simulink model "mainV03_52"  (R2016b)
settings: Solver=FixedStepAuto  StartTime=0.0  StopTime=inf  FixedStep=Ts  MaxStep=0.2  RelTol=1e-2
undefined symbols (not defined in the file): checks, datetime, decyear, delta_e, deltae_degrees, deltafl_degrees, deltafr_degrees, deltar_degrees, deltat_1, deltat_2, deltat_3, deltat_4, deltat_5, Earth, F, ft, groundReaction, initialValues, juliandate, LD, leapyear, Light, m, MIL, Newton, Raphson, s, sigbuilder_block, Ts, WGS84
libraries: simulink x27, aerolibutil x17, aerolibtransform2 x12, aerolibasang x5, aerolib6dofsys x5, aerolib6dof2 x4, aerolibwind2 x3, aerolibbdyn x3, aerolibconvert2 x3, aerolibactuator x2, aerolibgravity2 x2, aerolibnav x2
(part 3 of 6)

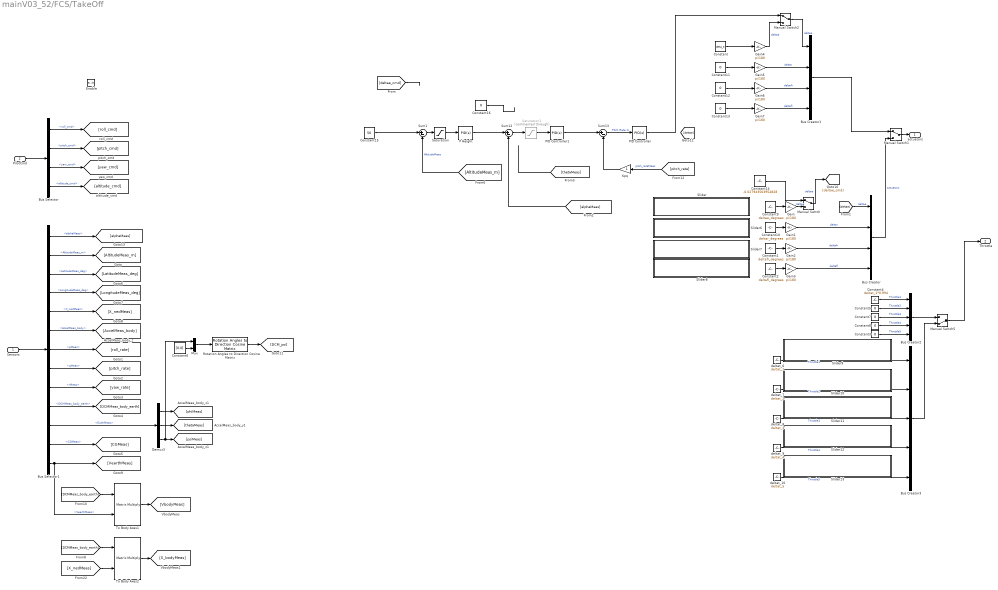
== system mainV03_52/FCS/TakeOff ==
  Sensors : Inport  OutDataTypeStr=Bus: SensorsBus
  PilotCmd : Inport  Port=2  OutDataTypeStr=Bus: CommandBus
  Enable : EnablePort
  Bus Creator : BusCreator  Inputs='deltae','deltar','deltafr','deltafl'  OutDataTypeStr=Bus: ActuatorsBus  NonVirtualBus=on
  Bus Creator1 : BusCreator  Inputs='deltae','deltar','deltafr','deltafl'  OutDataTypeStr=Bus: ActuatorsBus  NonVirtualBus=on
  Bus Creator2 : BusCreator  Inputs='Throttle1','Throttle2','Throttle3','Throttle4','Throttle5'  OutDataTypeStr=Bus: ThrottleBus  NonVirtualBus=on
  Bus Creator3 : BusCreator  Inputs='Throttle1','Throttle2','Throttle3','Throttle4','Throttle5'  OutDataTypeStr=Bus: ThrottleBus  NonVirtualBus=on
  Bus Selector : BusSelector  OutputSignals=roll_cmd,pitch_cmd,yaw_cmd,altitude_cmd
  Bus Selector1 : BusSelector  OutputSignals=alphaMeas,LLAMeas.AltitudeMeas_m,LLAMeas.LatitudeMeas_deg,LLAMeas.LongitudeMeas_deg,X_nedMeas,AccelMeas_body,OmegaMeas_body.pMeas,OmegaMeas_body.qMeas,OmegaMeas_body.rMeas,DCMMeas_body_earth,EulerMeas,CGMeas,VearthMeas
  Constant : Constant  Value=delta_e
  Constant1 : Constant  Value=deltafr_degrees
  Constant10 : Constant  Value=deltar_degrees
  Constant{3,5,7..8,11..13,16} (8 alike) : Constant  Value=0
  Constant14 : Constant  Value=-0.027943563954828
  Constant15 : Constant  Value=50
  Constant2 : Constant  Value=deltafl_degrees
  Constant4 : Constant  Value=deltat_1*0.994
  Constant6 : Constant  Value=[0,0]
  Constant9 : Constant  Value=deltae_degrees
  Demux3 : Demux  Outputs=3
  Gain{,1..7} (8 alike) : Gain  Gain=pi/180
  Kpq : Gain
  Manual Switch : ManualSwitch
  Manual Switch1 : ManualSwitch
  Manual Switch2 : ManualSwitch
  Manual Switch5 : ManualSwitch  CurrentSetting=0
  Mux : Mux  Inputs=2
  P Height : simulink/Continuous/PID Controller  Controller=PID  TimeDomain=Continuous-time  SampleTime=-1  IntegratorMethod=Forward Euler  FilterMethod=Forward Euler  Form=Parallel  UseFilter=on  ControllerParametersSource=internal  P=0.1  I=0  D=0.3  N=100  InitialConditionSource=internal  InitialConditionForIntegrator=0  InitialConditionForFilter=0  ExternalReset=none  LimitOutput=on  UpperSaturationLimit=10*pi/180  LowerSaturationLimit=-10*pi/180  LinearizeAsGain=on  AntiWindupMode=none  Kb=1  TrackingMode=off  Kt=1  PParamMin=[]  PParamMax=[]  IParamMin=[]  IParamMax=[]  DParamMin=[]  DParamMax=[]  NParamMin=[]  NParamMax=[]  KbParamMin=[]  KbParamMax=[]  KtParamMin=[]  KtParamMax=[]  POutMin=[]  POutMax=[]  IOutMin=[]  IOutMax=[]  DOutMin=[]  DOutMax=[]  NOutMin=[]  NOutMax=[]  KbOutMin=[]  KbOutMax=[]  KtOutMin=[]  KtOutMax=[]  IntegratorOutMin=[]  IntegratorOutMax=[]  FilterOutMin=[]  FilterOutMax=[]  SumOutMin=[]  SumOutMax=[]  SumI1OutMin=[]  SumI1OutMax=[]  SumI2OutMin=[]  SumI2OutMax=[]  SumI3OutMin=[]  SumI3OutMax=[]  SumDOutMin=[]  SumDOutMax=[]  SaturationOutMin=[]  SaturationOutMax=[]  IntegratorContinuousStateAttributes=''  IntegratorStateMustResolveToSignalObject=off  IntegratorRTWStateStorageClass=Auto  FilterContinuousStateAttributes=''  FilterStateMustResolveToSignalObject=off  FilterRTWStateStorageClass=Auto  DifferentiatorICPrevScaledInput=0  DifferentiatorOutMin=[]  DifferentiatorOutMax=[]
  PID Controller : simulink/Continuous/PID Controller  Controller=PID  TimeDomain=Continuous-time  SampleTime=-1  IntegratorMethod=Forward Euler  FilterMethod=Forward Euler  Form=Parallel  UseFilter=on  ControllerParametersSource=internal  P=-20  I=0  D=0  N=100  InitialConditionSource=internal  InitialConditionForIntegrator=0  InitialConditionForFilter=0  ExternalReset=none  LimitOutput=on  UpperSaturationLimit=40*pi/180  LowerSaturationLimit=-40*pi/180  LinearizeAsGain=on  AntiWindupMode=none  Kb=1  TrackingMode=off  Kt=1  PParamMin=[]  PParamMax=[]  IParamMin=[]  IParamMax=[]  DParamMin=[]  DParamMax=[]  NParamMin=[]  NParamMax=[]  KbParamMin=[]  KbParamMax=[]  KtParamMin=[]  KtParamMax=[]  POutMin=[]  POutMax=[]  IOutMin=[]  IOutMax=[]  DOutMin=[]  DOutMax=[]  NOutMin=[]  NOutMax=[]  KbOutMin=[]  KbOutMax=[]  KtOutMin=[]  KtOutMax=[]  IntegratorOutMin=[]  IntegratorOutMax=[]  FilterOutMin=[]  FilterOutMax=[]  SumOutMin=[]  SumOutMax=[]  SumI1OutMin=[]  SumI1OutMax=[]  SumI2OutMin=[]  SumI2OutMax=[]  SumI3OutMin=[]  SumI3OutMax=[]  SumDOutMin=[]  SumDOutMax=[]  SaturationOutMin=[]  SaturationOutMax=[]  IntegratorContinuousStateAttributes=''  IntegratorStateMustResolveToSignalObject=off  IntegratorRTWStateStorageClass=Auto  FilterContinuousStateAttributes=''  FilterStateMustResolveToSignalObject=off  FilterRTWStateStorageClass=Auto  DifferentiatorICPrevScaledInput=0  DifferentiatorOutMin=[]  DifferentiatorOutMax=[]
  PID Controller1 : simulink/Continuous/PID Controller  Controller=PID  TimeDomain=Continuous-time  SampleTime=-1  IntegratorMethod=Forward Euler  FilterMethod=Forward Euler  Form=Parallel  UseFilter=on  ControllerParametersSource=internal  P=10  I=0  D=0  N=100  InitialConditionSource=internal  InitialConditionForIntegrator=0  InitialConditionForFilter=0  ExternalReset=none  LimitOutput=off  UpperSaturationLimit=inf  LowerSaturationLimit=-inf  LinearizeAsGain=on  AntiWindupMode=none  Kb=1  TrackingMode=off  Kt=1  PParamMin=[]  PParamMax=[]  IParamMin=[]  IParamMax=[]  DParamMin=[]  DParamMax=[]  NParamMin=[]  NParamMax=[]  KbParamMin=[]  KbParamMax=[]  KtParamMin=[]  KtParamMax=[]  POutMin=[]  POutMax=[]  IOutMin=[]  IOutMax=[]  DOutMin=[]  DOutMax=[]  NOutMin=[]  NOutMax=[]  KbOutMin=[]  KbOutMax=[]  KtOutMin=[]  KtOutMax=[]  IntegratorOutMin=[]  IntegratorOutMax=[]  FilterOutMin=[]  FilterOutMax=[]  SumOutMin=[]  SumOutMax=[]  SumI1OutMin=[]  SumI1OutMax=[]  SumI2OutMin=[]  SumI2OutMax=[]  SumI3OutMin=[]  SumI3OutMax=[]  SumDOutMin=[]  SumDOutMax=[]  SaturationOutMin=[]  SaturationOutMax=[]  IntegratorContinuousStateAttributes=''  IntegratorStateMustResolveToSignalObject=off  IntegratorRTWStateStorageClass=Auto  FilterContinuousStateAttributes=''  FilterStateMustResolveToSignalObject=off  FilterRTWStateStorageClass=Auto  DifferentiatorICPrevScaledInput=0  DifferentiatorOutMin=[]  DifferentiatorOutMax=[]
  Rotation Angles to Direction Cosine Matrix : aerolibtransform2/Rotation Angles to Direction Cosine Matrix  rotationOrder=ZYX
  Saturation : Saturate  UpperLimit=25  LowerLimit=-25
  Saturation1 : Saturate  Commented=through  UpperLimit=10*pi/180  LowerLimit=-10*pi/180
  Slider : Subsystem  DialogController=hmiCreateDDGDialog  IsWebBlock=on  mask(MWDashboardBlock){webBlockId=9a8c1f82-5c06-438c-a725-2b399ee2535c, webBlockType=slider, ShowInLibBrowser=on, ShowInitialText=on, HMISrcModelName=mainV03_52}
      mask prompts: webBlockId "WebBlock Id"; webBlockType "WebBlock Type"; HMISrcModelName "Source Model"
      mask help: SimulinkHMI:dialogs:SliderDialogDesc
      mask Help: helpview([docroot '/mapfiles/simulink.map'], 'hmi_slider')
      mask Display:
      | if strcmp(get_param(bdroot(gcb),'BlockDiagramType'), 'library')
      |     image([(matlabroot) '/toolbox/simulink/hmi/icons/Slider.png']);
      | end
  Slider10 : Subsystem  DialogController=hmiCreateDDGDialog  IsWebBlock=on  mask(MWDashboardBlock){webBlockId=a6acb658-825e-439a-aa71-b8e8fe67d03f, webBlockType=slider, ShowInLibBrowser=on, ShowInitialText=on, HMISrcModelName=mainV03_52}
      mask prompts: webBlockId "WebBlock Id"; webBlockType "WebBlock Type"; HMISrcModelName "Source Model"
      mask help: SimulinkHMI:dialogs:SliderDialogDesc
      mask Help: helpview([docroot '/mapfiles/simulink.map'], 'hmi_slider')
      mask Display:
      | if strcmp(get_param(bdroot(gcb),'BlockDiagramType'), 'library')
      |     image([(matlabroot) '/toolbox/simulink/hmi/icons/Slider.png']);
      | end
  Slider11 : Subsystem  DialogController=hmiCreateDDGDialog  IsWebBlock=on  mask(MWDashboardBlock){webBlockId=02c5b359-6bb3-4adf-954f-3b6b7255ea2c, webBlockType=slider, ShowInLibBrowser=on, ShowInitialText=on, HMISrcModelName=mainV03_52}
      mask prompts: webBlockId "WebBlock Id"; webBlockType "WebBlock Type"; HMISrcModelName "Source Model"
      mask help: SimulinkHMI:dialogs:SliderDialogDesc
      mask Help: helpview([docroot '/mapfiles/simulink.map'], 'hmi_slider')
      mask Display:
      | if strcmp(get_param(bdroot(gcb),'BlockDiagramType'), 'library')
      |     image([(matlabroot) '/toolbox/simulink/hmi/icons/Slider.png']);
      | end
  Slider12 : Subsystem  DialogController=hmiCreateDDGDialog  IsWebBlock=on  mask(MWDashboardBlock){webBlockId=a5024071-52bc-4797-a61b-30869e68ef58, webBlockType=slider, ShowInLibBrowser=on, ShowInitialText=on, HMISrcModelName=mainV03_52}
      mask prompts: webBlockId "WebBlock Id"; webBlockType "WebBlock Type"; HMISrcModelName "Source Model"
      mask help: SimulinkHMI:dialogs:SliderDialogDesc
      mask Help: helpview([docroot '/mapfiles/simulink.map'], 'hmi_slider')
      mask Display:
      | if strcmp(get_param(bdroot(gcb),'BlockDiagramType'), 'library')
      |     image([(matlabroot) '/toolbox/simulink/hmi/icons/Slider.png']);
      | end
  Slider13 : Subsystem  DialogController=hmiCreateDDGDialog  IsWebBlock=on  mask(MWDashboardBlock){webBlockId=84f9b1f8-c67e-4667-9ecb-89bd91a4d659, webBlockType=slider, ShowInLibBrowser=on, ShowInitialText=on, HMISrcModelName=mainV03_52}
      mask prompts: webBlockId "WebBlock Id"; webBlockType "WebBlock Type"; HMISrcModelName "Source Model"
      mask help: SimulinkHMI:dialogs:SliderDialogDesc
      mask Help: helpview([docroot '/mapfiles/simulink.map'], 'hmi_slider')
      mask Display:
      | if strcmp(get_param(bdroot(gcb),'BlockDiagramType'), 'library')
      |     image([(matlabroot) '/toolbox/simulink/hmi/icons/Slider.png']);
      | end
  Slider6 : Subsystem  DialogController=hmiCreateDDGDialog  IsWebBlock=on  mask(MWDashboardBlock){webBlockId=89a52f80-8c90-4f33-b6a7-43d087fc50d5, webBlockType=slider, ShowInLibBrowser=on, ShowInitialText=on, HMISrcModelName=mainV03_52}
      mask prompts: webBlockId "WebBlock Id"; webBlockType "WebBlock Type"; HMISrcModelName "Source Model"
      mask help: SimulinkHMI:dialogs:SliderDialogDesc
      mask Help: helpview([docroot '/mapfiles/simulink.map'], 'hmi_slider')
      mask Display:
      | if strcmp(get_param(bdroot(gcb),'BlockDiagramType'), 'library')
      |     image([(matlabroot) '/toolbox/simulink/hmi/icons/Slider.png']);
      | end
  Slider7 : Subsystem  DialogController=hmiCreateDDGDialog  IsWebBlock=on  mask(MWDashboardBlock){webBlockId=bc2a720f-239d-4f19-b3ff-3602adab8c3e, webBlockType=slider, ShowInLibBrowser=on, ShowInitialText=on, HMISrcModelName=mainV03_52}
      mask prompts: webBlockId "WebBlock Id"; webBlockType "WebBlock Type"; HMISrcModelName "Source Model"
      mask help: SimulinkHMI:dialogs:SliderDialogDesc
      mask Help: helpview([docroot '/mapfiles/simulink.map'], 'hmi_slider')
      mask Display:
      | if strcmp(get_param(bdroot(gcb),'BlockDiagramType'), 'library')
      |     image([(matlabroot) '/toolbox/simulink/hmi/icons/Slider.png']);
      | end
  Slider8 : Subsystem  DialogController=hmiCreateDDGDialog  IsWebBlock=on  mask(MWDashboardBlock){webBlockId=e103cd05-37e1-4625-b96a-48a5402d1310, webBlockType=slider, ShowInLibBrowser=on, ShowInitialText=on, HMISrcModelName=mainV03_52}
      mask prompts: webBlockId "WebBlock Id"; webBlockType "WebBlock Type"; HMISrcModelName "Source Model"
      mask help: SimulinkHMI:dialogs:SliderDialogDesc
      mask Help: helpview([docroot '/mapfiles/simulink.map'], 'hmi_slider')
      mask Display:
      | if strcmp(get_param(bdroot(gcb),'BlockDiagramType'), 'library')
      |     image([(matlabroot) '/toolbox/simulink/hmi/icons/Slider.png']);
      | end
  Slider9 : Subsystem  DialogController=hmiCreateDDGDialog  IsWebBlock=on  mask(MWDashboardBlock){webBlockId=3e784728-11ac-4915-a19c-d9ef06d9d826, webBlockType=slider, ShowInLibBrowser=on, ShowInitialText=on, HMISrcModelName=mainV03_52}
      mask prompts: webBlockId "WebBlock Id"; webBlockType "WebBlock Type"; HMISrcModelName "Source Model"
      mask help: SimulinkHMI:dialogs:SliderDialogDesc
      mask Help: helpview([docroot '/mapfiles/simulink.map'], 'hmi_slider')
      mask Display:
      | if strcmp(get_param(bdroot(gcb),'BlockDiagramType'), 'library')
      |     image([(matlabroot) '/toolbox/simulink/hmi/icons/Slider.png']);
      | end
  Sum1 : Sum  Inputs=|+-
  Sum12 : Sum  Inputs=|+-
  Sum13 : Sum  Inputs=|+-
  To Body Axes1 : Product  Multiplication=Matrix(*)  SaturateOnIntegerOverflow=on  InputSameDT=on  OutDataTypeStr=Inherit: Same as first input
  To Body Axes2 : Product  Multiplication=Matrix(*)  SaturateOnIntegerOverflow=on  InputSameDT=on  OutDataTypeStr=Inherit: Same as first input
  deltat_10 : Constant  Value=deltat_5
  deltat_6 : Constant  Value=deltat_1
  deltat_7 : Constant  Value=deltat_2
  deltat_8 : Constant  Value=deltat_3
  deltat_9 : Constant  Value=deltat_4
  actuators : Outport
  Throttle : Outport  Port=2  OutDataTypeStr=Bus: ThrottleBus
  wires:
  PilotCmd/1 -> Bus Selector/1
  Sensors/1 -> Bus Selector1/1
  Bus Selector1/2 -> [AltitudeMeas_m]  "<AltitudeMeas_m>"
  Bus Selector/1 -> [roll_cmd]  "<roll_cmd>"
  Bus Selector/2 -> [pitch_cmd]  "<pitch_cmd>"
  Bus Selector/3 -> [yaw_cmd]  "<yaw_cmd>"
  Bus Selector/4 -> [altitude_cmd]  "<altitude_cmd>"
  Bus Selector1/7 -> [roll_rate]  "<pMeas>"
  Bus Selector1/8 -> [pitch_rate]  "<qMeas>"
  Bus Selector1/9 -> [yaw_rate]  "<rMeas>"
  Bus Selector1/10 -> [DCMMeas_body_earth]  "<DCMMeas_body_earth>"
  Demux3/1 -> [phiMeas]
  Demux3/2 -> [thetaMeas]
  Demux3/3 -> Mux/1, [psiMeas]
  Bus Selector1/12 -> [CGMeas]  "<CGMeas>"
  Bus Selector1/3 -> [LatitudeMeas_deg]  "<LatitudeMeas_deg>"
  Bus Selector1/4 -> [LongitudeMeas_deg]  "<LongitudeMeas_deg>"
  Bus Selector1/6 -> [AccelMeas_body]  "<AccelMeas_body>"
  Bus Selector1/5 -> [X_nedMeas]  "<X_nedMeas>"
  Bus Selector1/13 -> To Body Axes1/2, [VearthMeas]  "<VearthMeas>"
  [DCMMeas_body_earth] -> To Body Axes1/1
  To Body Axes1/1 -> [VbodyMeas]
  To Body Axes2/1 -> [X_bodyMeas]
  [DCMMeas_body_earth] -> To Body Axes2/1
  [X_nedMeas] -> To Body Axes2/2
  Bus Selector1/11 -> Demux3/1  "<EulerMeas>"
  Constant6/1 -> Mux/2
  Mux/1 -> Rotation Angles to Direction Cosine Matrix/1
  Rotation Angles to Direction Cosine Matrix/1 -> [DCM_psi]
  Bus Creator/1 -> Manual Switch1/2  "actuators"
  Gain1/1 -> Bus Creator/2  "deltar"
  Gain2/1 -> Bus Creator/3  "deltafr"
  Gain3/1 -> Bus Creator/4  "deltafl"
  Manual Switch/1 -> [deltae_cmd]  "deltae"
  Constant10/1 -> Gain1/1
  Constant1/1 -> Gain2/1
  Constant2/1 -> Gain3/1
  Constant4/1 -> Bus Creator2/1  "Throttle1"
  Constant7/1 -> Bus Creator2/3  "Throttle3"
  Constant5/1 -> Bus Creator2/2  "Throttle2"
  Constant8/1 -> Bus Creator2/4  "Throttle4"
  Constant3/1 -> Bus Creator2/5  "Throttle5"
  deltat_6/1 -> Bus Creator3/1  "Throttle1"
  deltat_8/1 -> Bus Creator3/3  "Throttle3"
  deltat_7/1 -> Bus Creator3/2  "Throttle2"
  deltat_9/1 -> Bus Creator3/4  "Throttle4"
  deltat_10/1 -> Bus Creator3/5  "Throttle5"
  Bus Creator2/1 -> Manual Switch5/1
  Bus Creator3/1 -> Manual Switch5/2
  Manual Switch5/1 -> Throttle/1
  Gain5/1 -> Bus Creator1/2  "deltar"
  Gain6/1 -> Bus Creator1/3  "deltafr"
  Gain7/1 -> Bus Creator1/4  "deltafl"
  Gain4/1 -> Manual Switch2/2  "deltae"
  Bus Creator1/1 -> Manual Switch1/1
  Manual Switch1/1 -> actuators/1
  Constant/1 -> Gain4/1
  Constant13/1 -> Gain7/1
  Constant12/1 -> Gain6/1
  Constant11/1 -> Gain5/1
  [pitch_rate] -> Kpq/1  "pitch_rateMeas"
  Sum1/1 -> Saturation/1
  Sum13/1 -> PID Controller/1  "Pitch Rate In"
  Sum12/1 -> Saturation1/1
  [AltitudeMeas_m] -> Sum1/2  "AltitudeMeas"
  P Height/1 -> Sum12/1
  Gain/1 -> Manual Switch/2  "deltae"
  [deltae_cmd] -> ?
  Kpq/1 -> Sum13/2
  [alphaMeas] -> Sum12/2
  Manual Switch2/1 -> Bus Creator1/1  "deltae"
  [deltae] -> Bus Creator/1  "deltae"
  Constant14/1 -> Manual Switch/1
  Constant9/1 -> Gain/1
  Bus Selector1/1 -> [alphaMeas]  "<alphaMeas>"
  Constant15/1 -> Sum1/1
  Constant16/1 -> ?
  PID Controller/1 -> Manual Switch2/1
  [thetaMeas] -> ?
  PID Controller1/1 -> Sum13/1
  Saturation/1 -> P Height/1
  Saturation1/1 -> PID Controller1/1

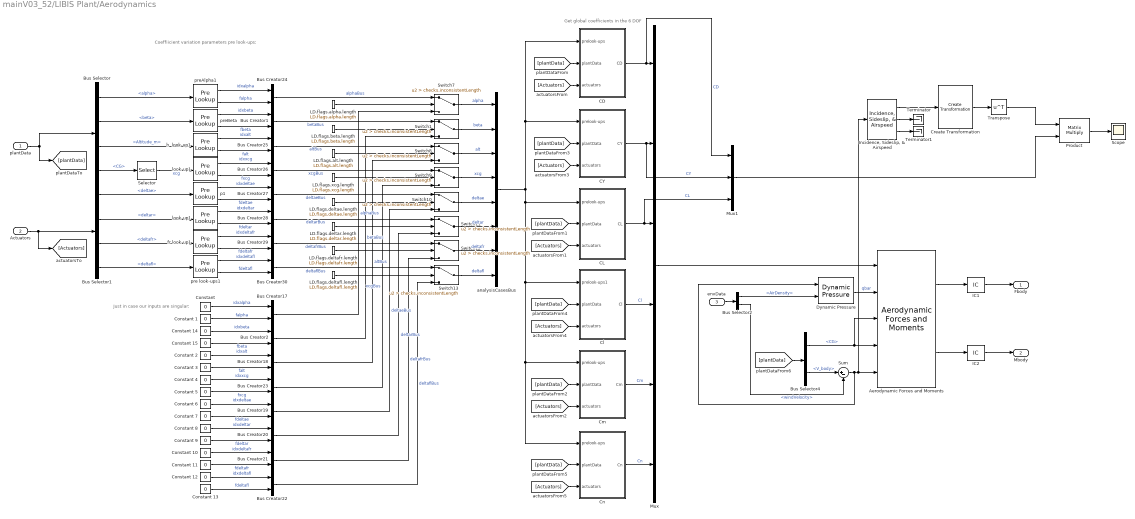
== system mainV03_52/LIBIS Plant/Aerodynamics ==
  note: Just in case our inputs are singular:
  note: Get global coefficients in the 6 DOF
  note: Coeffiicient variation parameters pre look-ups:
  plantData : Inport
  Actuators : Inport  Port=2  OutDataTypeStr=Bus: ActuatorsBus
  envData : Inport  Port=3
  " look-up1" : PreLookup  BreakpointsData=LD.xcg  BeginIndexSearchUsingPreviousIndexResult=on  UseLastBreakpoint=on  IndexDataTypeStr=int32  FractionDataTypeStr=double
  "Aerodynamic Forces and Moments " : aerolibadyn/Aerodynamic Forces and Moments   inputAxes=Stability  outputForceAxes=Body  outputMomentAxes=Body  S=LD.sref  b=LD.blref  cbar=LD.cbar
  Bus Creator1 : BusCreator  Inputs='idxbeta','fbeta'  OutDataTypeStr=Bus: betaBus  NonVirtualBus=on
  Bus Creator17 : BusCreator  Inputs='idxalpha','falpha'  OutDataTypeStr=Bus: alphaBus  NonVirtualBus=on
  Bus Creator18 : BusCreator  Inputs='idxalt','falt'  OutDataTypeStr=Bus: altBus  NonVirtualBus=on
  Bus Creator19 : BusCreator  Inputs='idxdeltae','fdeltae'  OutDataTypeStr=Bus: deltaeBus  NonVirtualBus=on
  Bus Creator2 : BusCreator  Inputs='idxbeta','fbeta'  OutDataTypeStr=Bus: betaBus  NonVirtualBus=on
  Bus Creator20 : BusCreator  Inputs='idxdeltar','fdeltar'  OutDataTypeStr=Bus: deltarBus  NonVirtualBus=on
  Bus Creator21 : BusCreator  Inputs='idxdeltafr','fdeltafr'  OutDataTypeStr=Bus: deltafrBus  NonVirtualBus=on
  Bus Creator22 : BusCreator  Inputs='idxdeltafl','fdeltafl'  OutDataTypeStr=Bus: deltaflBus  NonVirtualBus=on
  Bus Creator23 : BusCreator  Inputs='idxxcg','fxcg'  OutDataTypeStr=Bus: xcgBus  NonVirtualBus=on
  Bus Creator24 : BusCreator  Inputs='idxalpha','falpha'  OutDataTypeStr=Bus: alphaBus  NonVirtualBus=on
  Bus Creator25 : BusCreator  Inputs='idxalt','falt'  OutDataTypeStr=Bus: altBus  NonVirtualBus=on
  Bus Creator26 : BusCreator  Inputs='idxxcg','fxcg'  OutDataTypeStr=Bus: xcgBus  NonVirtualBus=on
  Bus Creator27 : BusCreator  Inputs='idxdeltae','fdeltae'  OutDataTypeStr=Bus: deltaeBus  NonVirtualBus=on
  Bus Creator28 : BusCreator  Inputs='idxdeltar','fdeltar'  OutDataTypeStr=Bus: deltarBus  NonVirtualBus=on
  Bus Creator29 : BusCreator  Inputs='idxdeltafr','fdeltafr'  OutDataTypeStr=Bus: deltafrBus  NonVirtualBus=on
  Bus Creator30 : BusCreator  Inputs='idxdeltafl','fdeltafl'  OutDataTypeStr=Bus: deltaflBus  NonVirtualBus=on
  Bus Selector : BusSelector  OutputSignals=alpha,beta,LLA.Altitude_m,CG
  Bus Selector1 : BusSelector  OutputSignals=deltae,deltar,deltafr,deltafl
  Bus Selector2 : BusSelector  OutputSignals=AirDensity,windVelocity
  Bus Selector4 : BusSelector  OutputSignals=CG,V_body
  CD : Subsystem
  CL : Subsystem
  CY : Subsystem
  Cl : Subsystem
  Cm : Subsystem
  Cn : Subsystem
  Constant {,2,4,6,8,10,12,14} (8 alike) : Constant  Value=0  OutDataTypeStr=int32
  Constant {1,3,5,7,9,11,13,15} (8 alike) : Constant  Value=0
  Create Transformation : aerolibadynsys/Stability to Body/Create Transformation
  Dynamic Pressure : aerolibasang/Dynamic Pressure
  IC1 : InitialCondition  Value=[0 0 0]
  IC2 : InitialCondition  Value=[0 0 0]
  "Incidence, Sideslip, & Airspeed" : aerolibasang/Incidence, Sideslip, & Airspeed
  LD.flags.alpha.length : Constant  Value=LD.flags.alpha.length
  LD.flags.alt.length : Constant  Value=LD.flags.alt.length
  LD.flags.beta.length : Constant  Value=LD.flags.beta.length
  LD.flags.deltae.length : Constant  Value=LD.flags.deltae.length
  LD.flags.deltafl.length : Constant  Value=LD.flags.deltafl.length
  LD.flags.deltafr.length : Constant  Value=LD.flags.deltafr.length
  LD.flags.deltar.length : Constant  Value=LD.flags.deltar.length
  LD.flags.xcg.length : Constant  Value=LD.flags.xcg.length
  Mux : Mux  Inputs=6
  Mux1 : Mux  Inputs=3
  Product : Product  Multiplication=Matrix(*)  RndMeth=Zero
  Scope : Scope
  Selector : Selector  InputPortWidth=3  IndexOptions=Index vector (dialog)  Indices=[1 ]  OutputSizes=1
  Sum : Sum  Inputs=|+-
  Switch{1,7..13} (8 alike) : Switch  Criteria=u2 > Threshold  Threshold=checks.inconsistentLength
  Terminator : Terminator
  Terminator1 : Terminator
  Transpose : Math  Operator=transpose  SaturateOnIntegerOverflow=on
  analysisCasesBus : BusCreator  Inputs='alpha','beta','alt','xcg','deltae','deltar','deltafr','deltafl'  OutDataTypeStr=Bus: analysisCasesBus  NonVirtualBus=on
  fr look-up1 : PreLookup  BreakpointsData=LD.deltafr  BeginIndexSearchUsingPreviousIndexResult=on  UseLastBreakpoint=on  IndexDataTypeStr=int32  FractionDataTypeStr=double
  h  look-up1 : PreLookup  BreakpointsData=LD.alt  BeginIndexSearchUsingPreviousIndexResult=on  UseLastBreakpoint=on  IndexDataTypeStr=int32  FractionDataTypeStr=double
  look-up1 : PreLookup  BreakpointsData=LD.deltar  BeginIndexSearchUsingPreviousIndexResult=on  UseLastBreakpoint=on  IndexDataTypeStr=int32  FractionDataTypeStr=double
  p1 : PreLookup  BreakpointsData=LD.deltae  BeginIndexSearchUsingPreviousIndexResult=on  UseLastBreakpoint=on  IndexDataTypeStr=int32  FractionDataTypeStr=double
  pre look-ups1 : PreLookup  BreakpointsData=LD.deltafl  BeginIndexSearchUsingPreviousIndexResult=on  UseLastBreakpoint=on  IndexDataTypeStr=int32  FractionDataTypeStr=double
  preAlpha1 : PreLookup  BreakpointsData=LD.alpha  BeginIndexSearchUsingPreviousIndexResult=on  UseLastBreakpoint=on  IndexDataTypeStr=int32  FractionDataTypeStr=double
  preBeta : PreLookup  BreakpointsData=LD.beta  BeginIndexSearchUsingPreviousIndexResult=on  UseLastBreakpoint=on  IndexDataTypeStr=int32  FractionDataTypeStr=double
  Fbody : Outport  Unit=N
  Mbody : Outport  Port=2  Unit=N*m
  wires:
  plantData/1 -> Bus Selector/1, [plantData]
  preAlpha1/2 -> Bus Creator24/2  "falpha"
  preAlpha1/1 -> Bus Creator24/1  "idxalpha"
  h  look-up1/2 -> Bus Creator25/2  "falt"
  h  look-up1/1 -> Bus Creator25/1  "idxalt"
  " look-up1"/1 -> Bus Creator26/1  "idxxcg"
  " look-up1"/2 -> Bus Creator26/2  "fxcg"
  p1/2 -> Bus Creator27/2  "fdeltae"
  p1/1 -> Bus Creator27/1  "idxdeltae"
  look-up1/2 -> Bus Creator28/2  "fdeltar"
  look-up1/1 -> Bus Creator28/1  "idxdeltar"
  fr look-up1/2 -> Bus Creator29/2  "fdeltafr"
  fr look-up1/1 -> Bus Creator29/1  "idxdeltafr"
  pre look-ups1/1 -> Bus Creator30/1  "idxdeltafl"
  pre look-ups1/2 -> Bus Creator30/2  "fdeltafl"
  LD.flags.alpha.length/1 -> Switch7/2
  Bus Creator24/1 -> Switch7/1  "alphaBus"
  LD.flags.alt.length/1 -> Switch8/2
  Bus Creator25/1 -> Switch8/1  "altBus"
  LD.flags.xcg.length/1 -> Switch9/2
  Bus Creator26/1 -> Switch9/1  "xcgBus"
  LD.flags.deltae.length/1 -> Switch10/2
  Bus Creator27/1 -> Switch10/1  "deltaeBus"
  LD.flags.deltar.length/1 -> Switch11/2
  Bus Creator28/1 -> Switch11/1  "deltarBus"
  LD.flags.deltafr.length/1 -> Switch12/2
  Bus Creator29/1 -> Switch12/1  "deltafrBus"
  LD.flags.deltafl.length/1 -> Switch13/2
  Bus Creator30/1 -> Switch13/1  "deltaflBus"
  Bus Creator17/1 -> Switch7/3  "alphaBus"
  Bus Creator18/1 -> Switch8/3  "altBus"
  Bus Creator23/1 -> Switch9/3  "xcgBus"
  Bus Creator19/1 -> Switch10/3  "deltaeBus"
  Bus Creator20/1 -> Switch11/3  "deltarBus"
  Bus Creator21/1 -> Switch12/3  "deltafrBus"
  Bus Creator22/1 -> Switch13/3  "deltaflBus"
  Switch7/1 -> analysisCasesBus/1  "alpha"
  Switch8/1 -> analysisCasesBus/3  "alt"
  Switch9/1 -> analysisCasesBus/4  "xcg"
  Switch10/1 -> analysisCasesBus/5  "deltae"
  Switch11/1 -> analysisCasesBus/6  "deltar"
  Switch12/1 -> analysisCasesBus/7  "deltafr"
  Switch13/1 -> analysisCasesBus/8  "deltafl"
  Constant 1/1 -> Bus Creator17/2  "falpha"
  "Constant "/1 -> Bus Creator17/1  "idxalpha"
  Constant 3/1 -> Bus Creator18/2  "falt"
  Constant 2/1 -> Bus Creator18/1  "idxalt"
  Constant 4/1 -> Bus Creator23/1  "idxxcg"
  Constant 5/1 -> Bus Creator23/2  "fxcg"
  Constant 7/1 -> Bus Creator19/2  "fdeltae"
  Constant 6/1 -> Bus Creator19/1  "idxdeltae"
  Constant 9/1 -> Bus Creator20/2  "fdeltar"
  Constant 8/1 -> Bus Creator20/1  "idxdeltar"
  Constant 11/1 -> Bus Creator21/2  "fdeltafr"
  Constant 10/1 -> Bus Creator21/1  "idxdeltafr"
  Constant 12/1 -> Bus Creator22/1  "idxdeltafl"
  Constant 13/1 -> Bus Creator22/2  "fdeltafl"
  analysisCasesBus/1 -> CL/1(prelook-ups), Cl/1(prelook-ups1), Cn/1(prelook-ups), Cm/1(prelook-ups), CD/1(prelook-ups), CY/1(prelook-ups)
  Bus Selector/1 -> preAlpha1/1  "<alpha>"
  Bus Selector/3 -> h  look-up1/1  "<Altitude_m>"
  Bus Selector/4 -> Selector/1  "<CG>"
  Selector/1 -> " look-up1"/1  "xcg"
  Actuators/1 -> [Actuators], Bus Selector1/1
  Bus Selector1/1 -> p1/1  "<deltae>"
  Bus Selector1/2 -> look-up1/1  "<deltar>"
  Bus Selector1/3 -> fr look-up1/1  "<deltafr>"
  Bus Selector1/4 -> pre look-ups1/1  "<deltafl>"
  [plantData] -> CD/2(plantData)
  [Actuators] -> CD/3(actuators)
  [plantData] -> CL/2(plantData)
  [plantData] -> Cm/2(plantData)
  [plantData] -> CY/2(plantData)
  [Actuators] -> CY/3(actuators)
  [plantData] -> Cl/2(plantData)
  [Actuators] -> Cl/3(actuators)
  [plantData] -> Cn/2(plantData)
  [Actuators] -> Cn/3(actuators)
  Cn/1(Cn) -> Mux/6  "Cn"
  Cl/1(Cl) -> Mux/4  "Cl"
  CL/1(CL) -> Mux1/3, Mux/3  "CL"
  CY/1(CY) -> Mux1/2, Mux/2  "CY"
  CD/1(CD) -> Mux1/1, Mux/1  "CD"
  Cm/1(Cm) -> Mux/5  "Cm"
  Mux/1 -> "Aerodynamic Forces and Moments "/1
  "Aerodynamic Forces and Moments "/1 -> IC1/1
  "Aerodynamic Forces and Moments "/2 -> IC2/1
  envData/1 -> Bus Selector2/1
  [plantData] -> Bus Selector4/1
  Bus Selector4/1 -> "Aerodynamic Forces and Moments "/3, "Aerodynamic Forces and Moments "/4  "<CG>"
  [Actuators] -> CL/3(actuators)
  [Actuators] -> Cm/3(actuators)
  IC1/1 -> Fbody/1
  IC2/1 -> Mbody/1
  Dynamic Pressure/1 -> "Aerodynamic Forces and Moments "/2  "qbar"
  Bus Selector2/1 -> Dynamic Pressure/2  "<AirDensity>"
  Bus Selector4/2 -> Sum/1  "<V_body>"
  Bus Selector2/2 -> Sum/2  "<windVelocity>"
  Sum/1 -> "Aerodynamic Forces and Moments "/5, "Incidence, Sideslip, & Airspeed"/1, Dynamic Pressure/1
  preBeta/2 -> Bus Creator1/2  "fbeta"
  preBeta/1 -> Bus Creator1/1  "idxbeta"
  Bus Creator1/1 -> Switch1/1  "betaBus"
  Bus Selector/2 -> preBeta/1  "<beta>"
  Switch1/1 -> analysisCasesBus/2  "beta"
  LD.flags.beta.length/1 -> Switch1/2
  Constant 15/1 -> Bus Creator2/2  "fbeta"
  Constant 14/1 -> Bus Creator2/1  "idxbeta"
  Bus Creator2/1 -> Switch1/3  "betaBus"
  Product/1 -> Scope/1
  Mux1/1 -> Product/2
  "Incidence, Sideslip, & Airspeed"/1 -> Create Transformation/1
  Create Transformation/1 -> Transpose/1
  Transpose/1 -> Product/1
  "Incidence, Sideslip, & Airspeed"/2 -> Terminator/1
  "Incidence, Sideslip, & Airspeed"/3 -> Terminator1/1

== system mainV03_52/LIBIS Plant/Custom Variable Mass 6DOF (Euler Angles) (propio) ==
  Forces : Inport  Unit=N  PortDimensions=3
  Moments : Inport  Port=2  Unit=N*m  PortDimensions=3
  m_dot : Inport  Port=3  Unit=kg/s
  mass : Inport  Port=4  Unit=kg
  I_dot : Inport  Port=5  Unit=kg*m^2/s  PortDimensions=[3 3]
  I : Inport  Port=6  Unit=kg*m^2  PortDimensions=[3 3]
  Vre : Inport  Port=7  Unit=m/s
  Calculate DCM & Euler Angles : aerolib6dofsys/DCM & Euler Angles (Euler)  SystemSampleTime=-1
  Calculate omega_dot : aerolib6dofsys/Calculate omega_dot  SystemSampleTime=-1
  "Determine Force, Mass & Inertia" : aerolib6dofsys/Mass & Inertia (custom)  SystemSampleTime=-1
  Disallow CGS : UnitConfiguration  UnitSystemsStr=English,SI,SI (extended)  AllowAllUnitSystems=off
  Out9 : Terminator
  Product : Product  Inputs=*/  SaturateOnIntegerOverflow=on  OutDataTypeStr=Inherit: Same as first input
  Reshape : Reshape  OutputDimensions=""
  Sum2 : Sum  Inputs=|++  SaturateOnIntegerOverflow=on
  Transpose : Math  Operator=transpose  SaturateOnIntegerOverflow=on
  Vbxw : aerolibutil/3x3 Cross Product
  Velocity Conversion : aerolib6dof2/6DOF (Euler Angles)/Velocity Conversion
  Velocity Conversion1 : aerolib6dof2/6DOF (Euler Angles)/Velocity Conversion1
  Velocity Conversion2 : aerolib6dof2/6DOF (Euler Angles)/Velocity Conversion2
  "p,q,r " : Integrator  InitialCondition=pm_0
  "transform to Inertial axes " : aerolib6dof2/6DOF (Euler Angles)/transform to Inertial axes   SystemSampleTime=-1
  ub,vb,wb : Integrator  InitialCondition=Vm_0
  xe,ye,ze : Integrator  InitialCondition=xme_0  UpperSaturationLimit=[inf, inf, initialValues.href]  LowerSaturationLimit=[-inf, -inf, -inf]
  Ve : Outport  Unit=m/s
  Xe : Outport  Port=2  Unit=m
  Euler : Outport  Port=3  Unit=rad
  DCM : Outport  Port=4  Unit=1
  Vb : Outport  Port=5  Unit=m/s
  p,q,r : Outport  Port=6  Unit=rad/s
  pdot,qdot,rdot : Outport  Port=7  Unit=rad/s^2
  Ab : Outport  Port=8  Unit=m/s^2  PortDimensions=3
  wires:
  Velocity Conversion1/1 -> Ve/1
  "Determine Force, Mass & Inertia"/2 -> Product/2
  Vre/1 -> Velocity Conversion2/1
  Calculate DCM & Euler Angles/1 -> DCM/1, Transpose/1
  Transpose/1 -> "transform to Inertial axes "/2
  Calculate DCM & Euler Angles/2 -> Euler/1
  "Determine Force, Mass & Inertia"/4 -> Out9/1
  "p,q,r "/1 -> Calculate DCM & Euler Angles/1, p,q,r/1, Vbxw/2, Calculate omega_dot/1
  xe,ye,ze/1 -> Xe/1
  Velocity Conversion/1 -> Vb/1
  I_dot/1 -> "Determine Force, Mass & Inertia"/6
  "transform to Inertial axes "/1 -> Velocity Conversion1/1, xe,ye,ze/1
  mass/1 -> "Determine Force, Mass & Inertia"/3
  Velocity Conversion2/1 -> "Determine Force, Mass & Inertia"/1
  "Determine Force, Mass & Inertia"/1 -> Product/1
  Forces/1 -> "Determine Force, Mass & Inertia"/2
  Moments/1 -> Calculate omega_dot/3
  Product/1 -> Sum2/1
  m_dot/1 -> "Determine Force, Mass & Inertia"/4
  ub,vb,wb/1 -> Vbxw/1, "transform to Inertial axes "/1, Velocity Conversion/1
  "Determine Force, Mass & Inertia"/3 -> Calculate omega_dot/2
  I/1 -> "Determine Force, Mass & Inertia"/5
  Sum2/1 -> Ab/1, ub,vb,wb/1
  Calculate omega_dot/1 -> pdot,qdot,rdot/1, "p,q,r "/1
  Vbxw/1 -> Reshape/1
  Reshape/1 -> Sum2/2

== system mainV03_52/LIBIS Plant/Incidence, Sideslip ==
  "u, v, w" : Inport
  Airspeed : Sqrt  AlgorithmType=Newton-Raphson  SaturateOnIntegerOverflow=on
  Constant : Constant  Value=0
  Incidence : Trigonometry  Operator=atan2
  Product : Product  Inputs=*/  SaturateOnIntegerOverflow=on  OutDataTypeStr=Inherit: Same as first input
  Sideslip : Trigonometry  Operator=asin
  Subsystem : aerolibasang/Incidence, Sideslip, & Airspeed/Subsystem
  Subsystem1 : aerolibasang/Incidence, Sideslip, & Airspeed/Subsystem1
  Switch : Switch  Criteria=u2 > Threshold
  dot : aerolibasang/Incidence, Sideslip, & Airspeed/dot
  Alpha : Outport  Unit=rad  InitialOutput=0
  Beta : Outport  Port=2  Unit=rad  InitialOutput=0
  wires:
  Subsystem/1 -> Incidence/1
  Subsystem1/1 -> Product/1
  dot/1 -> Airspeed/1
  Airspeed/1 -> Switch/2, Product/2
  "u, v, w"/1 -> Subsystem/1, Subsystem1/1, dot/1
  Sideslip/1 -> Beta/1
  Product/1 -> Switch/1
  Switch/1 -> Sideslip/1
  Constant/1 -> Switch/3
  Subsystem/2 -> Incidence/2
  Incidence/1 -> Alpha/1

== system mainV03_52/LIBIS Plant/Inertia Block ==
  Estimate Center of Gravity : aerolibbdyn/Estimate Center of Gravity  fmass=LD.Inertia.fullMass  emass=LD.Inertia.emptyMass-1  fcg=LD.Inertia.fullCG  ecg=LD.Inertia.emptyCG
  Ixx : Constant  Value=LD.Inertia.Ixx
  Ixy : Constant  Value=LD.Inertia.Ixy
  Ixz : Constant  Value=LD.Inertia.Ixz
  Iyy : Constant  Value=LD.Inertia.Iyy
  Iyz : Constant  Value=LD.Inertia.Iyz
  Izz : Constant  Value=LD.Inertia.Izz
  Mux : Mux  Inputs=3
  Reshape : Reshape
  Symmetric Inertia Tensor : aerolibbdyn/Symmetric Inertia Tensor
  Symmetric Inertia Tensor1 : aerolibbdyn/Symmetric Inertia Tensor
  Vre_x (m/s) : Constant  Value=LD.Inertia.dmassdxb
  Vre_y (m/s) : Constant  Value=LD.Inertia.dmassdyb
  Vre_z (m/s) : Constant  Value=LD.Inertia.dmassdzb
  dIxx/dt : Constant  Value=LD.Inertia.dIxx
  dIxy/dt : Constant  Value=LD.Inertia.dIxy
  dIxz/dt : Constant  Value=LD.Inertia.dIxz
  dIyy/dt : Constant  Value=LD.Inertia.dIyy
  dIyz/dt : Constant  Value=LD.Inertia.dIyz
  dIzz/dt : Constant  Value=LD.Inertia.dIzz
  dmass/dt (kg/s) : Constant  Value=LD.Inertia.dmass
  mass (kg) : Constant  Value=LD.Inertia.mass
  dm/dt (kg/s) : Outport  Unit=kg/s
  m (kg) : Outport  Port=2  Unit=kg
  dI/dt (kg-m^2/s) : Outport  Port=3  Unit=kg*meter^2/s
  I (kg-m^2) : Outport  Port=4  Unit=kg*meter*meter
  Vre (m/s) : Outport  Port=5  Unit=meter/s
  CG : Outport  Port=6
  dCG/dt : Outport  Port=7
  wires:
  Symmetric Inertia Tensor/1 -> I (kg-m^2)/1  "I (kg-m^2)"
  Symmetric Inertia Tensor1/1 -> dI/dt (kg-m^2/s)/1  "dI/dt (kg-m^2/s)"
  dIxx/dt/1 -> Symmetric Inertia Tensor1/1  "dIxx/dt (kg-m^2/s)"
  dIxz/dt/1 -> Symmetric Inertia Tensor1/3  "dIxz/dt (kg-m^2/s)"
  dIxy/dt/1 -> Symmetric Inertia Tensor1/2  "dIxy/dt (kg-m^2/s)"
  dIyy/dt/1 -> Symmetric Inertia Tensor1/4  "dIyy/dt (kg-m^2/s)"
  dIzz/dt/1 -> Symmetric Inertia Tensor1/6  "dIzz/dt (kg-m^2/s)"
  dIyz/dt/1 -> Symmetric Inertia Tensor1/5  "dIyz/dt (kg-m^2/s)"
  Ixx/1 -> Symmetric Inertia Tensor/1  "Ixx (kg-m^2)"
  Ixz/1 -> Symmetric Inertia Tensor/3  "Ixz (kg-m^2)"
  Ixy/1 -> Symmetric Inertia Tensor/2  "Ixy (kg-m^2)"
  Iyy/1 -> Symmetric Inertia Tensor/4  "Iyy (kg-m^2)"
  Izz/1 -> Symmetric Inertia Tensor/6  "Izz (kg-m^2)"
  Iyz/1 -> Symmetric Inertia Tensor/5  "Iyz (kg-m^2)"
  mass (kg)/1 -> Estimate Center of Gravity/1, m (kg)/1  "m (kg)"
  dmass/dt (kg/s)/1 -> Estimate Center of Gravity/2, dm/dt (kg/s)/1  "dm/dt (kg/s)"
  Vre_x (m/s)/1 -> Mux/1  "Vre_x (m/s)"
  Vre_z (m/s)/1 -> Mux/3  "Vre_z (m/s)"
  Vre_y (m/s)/1 -> Mux/2  "Vre_y (m/s)"
  Mux/1 -> Vre (m/s)/1  "Vre (m/s)"
  Estimate Center of Gravity/1 -> Reshape/1  "CG"
  Estimate Center of Gravity/2 -> dCG/dt/1  "dCG/dt"
  Reshape/1 -> CG/1

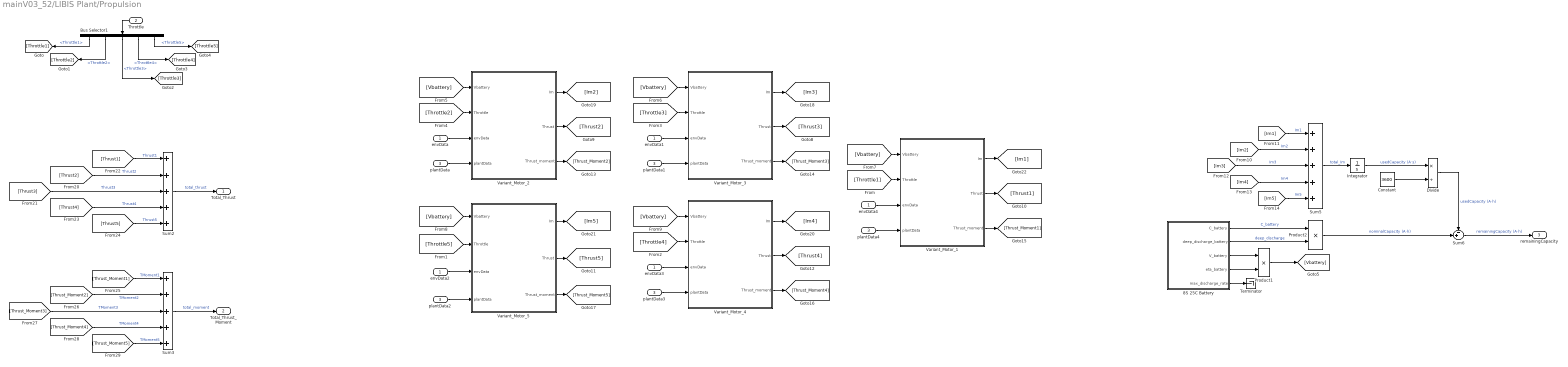
== system mainV03_52/LIBIS Plant/Propulsion ==
  envData : Inport
  Throttle : Inport  Port=2
  plantData : Inport  Port=3
  8S 25C Battery : Subsystem
  Bus Selector1 : BusSelector  OutputSignals=Throttle1,Throttle2,Throttle3,Throttle4,Throttle5
  Constant : Constant  Value=3600
  Divide : Product  Inputs=*/
  Integrator : Integrator
  Product1 : Product
  Product2 : Product
  Sum2 : Sum  Inputs=+++++
  Sum3 : Sum  Inputs=+++++
  Sum5 : Sum  Inputs=+++++
  Sum6 : Sum  Inputs=-+|
  Terminator : Terminator
  Variant_Motor_1 : Subsystem  Variant=on
      mask Display:
      | imageName='LIBIS_Motor1.png';
      | currentPath=get_param(bdroot, 'FileName');
      | positions=strfind(currentPath,'\');
      | imagePath=strcat(currentPath(1:positions(end-1)),'graphics\',imageName);
      | image(imagePath);
  Variant_Motor_2 : Subsystem  Variant=on
      mask Display:
      | imageName='LIBIS_Motor2.png';
      | currentPath=get_param(bdroot, 'FileName');
      | positions=strfind(currentPath,'\');
      | imagePath=strcat(currentPath(1:positions(end-1)),'graphics\',imageName);
      | image(imagePath);
  Variant_Motor_3 : Subsystem  Variant=on
      mask Display:
      | imageName='LIBIS_Motor3.png';
      | currentPath=get_param(bdroot, 'FileName');
      | positions=strfind(currentPath,'\');
      | imagePath=strcat(currentPath(1:positions(end-1)),'graphics\',imageName);
      | image(imagePath);
  Variant_Motor_4 : Subsystem  Variant=on
      mask Display:
      | imageName='LIBIS_Motor4.png';
      | currentPath=get_param(bdroot, 'FileName');
      | positions=strfind(currentPath,'\');
      | imagePath=strcat(currentPath(1:positions(end-1)),'graphics\',imageName);
      | image(imagePath);
  Variant_Motor_5 : Subsystem  Variant=on
      mask Display:
      | imageName='LIBIS_Motor5.png';
      | currentPath=get_param(bdroot, 'FileName');
      | positions=strfind(currentPath,'\');
      | imagePath=strcat(currentPath(1:positions(end-1)),'graphics\',imageName);
      | image(imagePath);
  envData{1..4} (4 alike) : InportShadow
  plantData{1..4} (4 alike) : InportShadow  Port=3
  Total_Thrust : Outport
  Total_Thrust_Moment : Outport  Port=2
  remainingCapacity : Outport  Port=3
  wires:
  Throttle/1 -> Bus Selector1/1
  Bus Selector1/1 -> [Throttle1]  "<Throttle1>"
  Bus Selector1/2 -> [Throttle2]  "<Throttle2>"
  Bus Selector1/3 -> [Throttle3]  "<Throttle3>"
  Bus Selector1/4 -> [Throttle4]  "<Throttle4>"
  Bus Selector1/5 -> [Throttle5]  "<Throttle5>"
  8S 25C Battery/3(V_battery) -> Product1/1
  8S 25C Battery/4(eta_battery) -> Product1/2
  8S 25C Battery/1(C_battery) -> Product2/1  "C_battery"
  8S 25C Battery/5(max_discharge_rate) -> Terminator/1
  8S 25C Battery/2(deep_discharge_battery) -> Product2/2  "deep_discharge"
  [Throttle5] -> Variant_Motor_5/2(Throttle)
  Variant_Motor_5/2(Thrust) -> [Thrust5]
  [Thrust1] -> Sum2/1  "Thrust1"
  [Thrust2] -> Sum2/2  "Thrust2"
  [Thrust3] -> Sum2/3  "Thrust3"
  [Thrust4] -> Sum2/4  "Thrust4"
  [Thrust5] -> Sum2/5  "Thrust5"
  Sum2/1 -> Total_Thrust/1  "total_thrust"
  Sum3/1 -> Total_Thrust_Moment/1  "total_moment"
  [Thrust_Moment1] -> Sum3/1  "TMoment1"
  [Thrust_Moment2] -> Sum3/2  "TMoment2"
  [Thrust_Moment3] -> Sum3/3  "TMoment3"
  [Thrust_Moment4] -> Sum3/4  "TMoment4"
  Variant_Motor_5/3(Thrust_moment) -> [Thrust_Moment5]
  [Thrust_Moment5] -> Sum3/5  "TMoment5"
  Product2/1 -> Sum6/2  "nominalCapacity (A·h)"
  Variant_Motor_5/1(Im) -> [Im5]
  [Im3] -> Sum5/3  "Im3"
  [Im2] -> Sum5/2  "Im2"
  [Im1] -> Sum5/1  "Im1"
  [Im4] -> Sum5/4  "Im4"
  [Im5] -> Sum5/5  "Im5"
  Sum5/1 -> Integrator/1  "total_Im"
  Sum6/1 -> remainingCapacity/1  "remainingCapacity (A·h)"
  Product1/1 -> [Vbattery]
  [Vbattery] -> Variant_Motor_5/1(Vbattery)
  Integrator/1 -> Divide/1  "usedCapacity (A·s)"
  Constant/1 -> Divide/2
  Divide/1 -> Sum6/1  "usedCapacity (A·h)"
  envData2/1 -> Variant_Motor_5/3(envData)
  plantData2/1 -> Variant_Motor_5/4(plantData)
  [Vbattery] -> Variant_Motor_2/1(Vbattery)
  [Throttle2] -> Variant_Motor_2/2(Throttle)
  Variant_Motor_2/1(Im) -> [Im2]
  Variant_Motor_2/2(Thrust) -> [Thrust2]
  Variant_Motor_2/3(Thrust_moment) -> [Thrust_Moment2]
  envData/1 -> Variant_Motor_2/3(envData)
  plantData/1 -> Variant_Motor_2/4(plantData)
  [Vbattery] -> Variant_Motor_3/1(Vbattery)
  [Throttle3] -> Variant_Motor_3/2(Throttle)
  Variant_Motor_3/3(Thrust_moment) -> [Thrust_Moment3]
  Variant_Motor_3/2(Thrust) -> [Thrust3]
  Variant_Motor_3/1(Im) -> [Im3]
  envData1/1 -> Variant_Motor_3/3(envData)
  plantData1/1 -> Variant_Motor_3/4(plantData)
  [Vbattery] -> Variant_Motor_4/1(Vbattery)
  [Throttle4] -> Variant_Motor_4/2(Throttle)
  Variant_Motor_4/1(Im) -> [Im4]
  Variant_Motor_4/2(Thrust) -> [Thrust4]
  Variant_Motor_4/3(Thrust_moment) -> [Thrust_Moment4]
  envData3/1 -> Variant_Motor_4/3(envData)
  plantData3/1 -> Variant_Motor_4/4(plantData)
  [Vbattery] -> Variant_Motor_1/1(Vbattery)
  [Throttle1] -> Variant_Motor_1/2(Throttle)
  Variant_Motor_1/1(Im) -> [Im1]
  Variant_Motor_1/2(Thrust) -> [Thrust1]
  Variant_Motor_1/3(Thrust_moment) -> [Thrust_Moment1]
  envData4/1 -> Variant_Motor_1/3(envData)
  plantData4/1 -> Variant_Motor_1/4(plantData)

== system mainV03_52/LIBIS Plant/Subsystem ==
  beta : Inport  Unit=rad
  alpha : Inport  Port=2  Unit=rad
  V_body : Inport  Port=3  Unit=meter/s
  Omega_body : Inport  Port=4  Unit=rad/s
  Accel_body : Inport  Port=5  Unit=m/s^2
  Constant1 : Constant  Value=0
  Constant11 : Constant  Value=0
  Direction Cosine Matrix Body to Wind : aerolibtransform2/Direction Cosine Matrix Body to Wind
  IC : InitialCondition  Value=0
  Mux4 : Mux  Inputs=2
  Product1 : Product  Multiplication=Matrix(*)  SaturateOnIntegerOverflow=on  InputSameDT=on  OutDataTypeStr=Inherit: Same as first input
  Selector : Selector  InputPortWidth=3  IndexOptions=Index vector (dialog)  Indices=[2]  OutputSizes=1
  Terminator : Terminator
  calc alpha_dot : Subsystem
  alpha_dot : Outport  Unit=rad/s
  beta_dot : Outport  Port=2
  wires:
  Direction Cosine Matrix Body to Wind/1 -> Product1/1
  Product1/1 -> calc alpha_dot/4(Vw)
  Mux4/1 -> Direction Cosine Matrix Body to Wind/1, calc alpha_dot/2(alpha,beta)
  Constant11/1 -> beta_dot/1  "beta_dot"
  alpha/1 -> Mux4/1
  Omega_body/1 -> Selector/1
  V_body/1 -> Product1/2
  Accel_body/1 -> calc alpha_dot/3(Ab)
  beta/1 -> Mux4/2
  calc alpha_dot/1(alpha_dot) -> IC/1
  Selector/1 -> calc alpha_dot/1(q)  "q"
  IC/1 -> Terminator/1
  Constant1/1 -> alpha_dot/1

== system mainV03_52/LIBIS Plant/TransferFunction ==
  In1 : Inport
  Demux4 : Demux  Outputs=3
  Mux1 : Mux  Inputs=3
  Transfer Fcn1 : TransferFcn  Denominator=[eps 1]
  Transfer Fcn4 : TransferFcn  Denominator=[eps 1]
  Transfer Fcn5 : TransferFcn  Denominator=[eps 1]
  Out1 : Outport
  wires:
  Transfer Fcn1/1 -> Mux1/1
  Transfer Fcn5/1 -> Mux1/3
  Mux1/1 -> Out1/1
  Demux4/2 -> Transfer Fcn4/1
  Transfer Fcn4/1 -> Mux1/2
  Demux4/1 -> Transfer Fcn1/1
  In1/1 -> Demux4/1
  Demux4/3 -> Transfer Fcn5/1

== system mainV03_52/LIBIS Plant/TransferFunctions ==
  In1 : Inport
  In2 : Inport  Port=2
  Demux : Demux  Outputs=3
  Demux1 : Demux  Outputs=3
  Mux : Mux  Inputs=3
  Mux1 : Mux  Inputs=3
  Transfer Fcn{,1..5} (6 alike) : TransferFcn  Denominator=[eps 1]
  Out1 : Outport
  Out2 : Outport  Port=2
  wires:
  Demux1/3 -> Transfer Fcn5/1
  Transfer Fcn3/1 -> Mux1/1
  In2/1 -> Demux1/1
  Transfer Fcn1/1 -> Mux/2
  Demux1/2 -> Transfer Fcn4/1
  Demux/1 -> Transfer Fcn/1
  Transfer Fcn4/1 -> Mux1/2
  Transfer Fcn2/1 -> Mux/3
  Transfer Fcn5/1 -> Mux1/3
  Transfer Fcn/1 -> Mux/1
  Demux/3 -> Transfer Fcn2/1
  Demux/2 -> Transfer Fcn1/1
  Mux1/1 -> Out2/1
  Demux1/1 -> Transfer Fcn3/1
  In1/1 -> Demux/1
  Mux/1 -> Out1/1

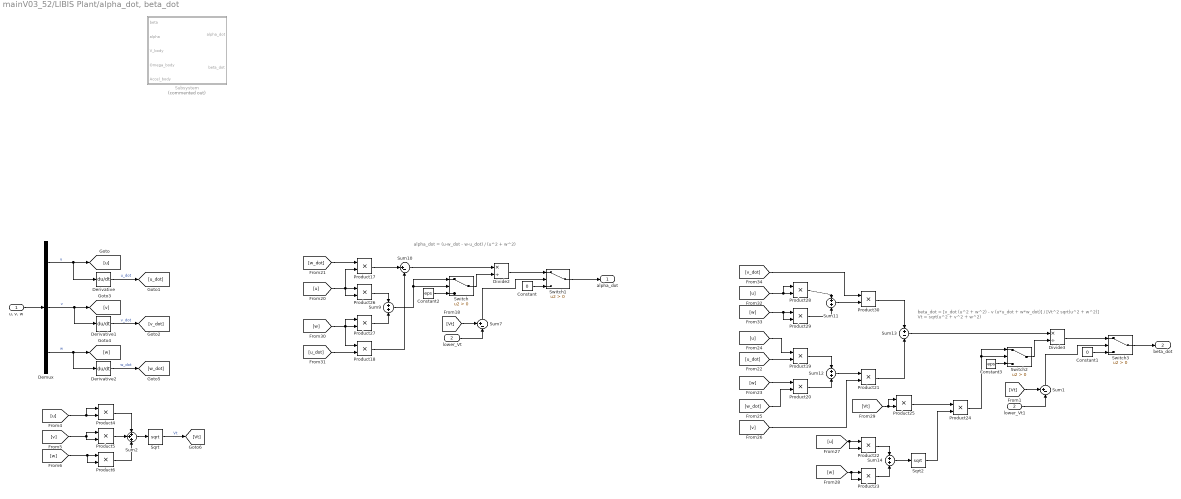
== system mainV03_52/LIBIS Plant/alpha_dot, beta_dot ==
  note: beta_dot = [v_dot (u^2 + w^2) - v (u*u_dot + w*w_dot)] / [Vt^2 sqrt(u^2 + w^2)]
      | Vt = sqrt(u^2 + v^2 + w^2)
  note: alpha_dot = (u·w_dot - w·u_dot) / (u^2 + w^2)
  "u, v, w" : Inport  Unit=meter/s
  lower_Vt : Inport  Port=2
  Constant : Constant  Value=0
  Constant1 : Constant  Value=0
  Constant2 : Constant  Value=eps
  Constant3 : Constant  Value=eps
  Demux : Demux  Outputs=3
  Derivative : Derivative
  Derivative1 : Derivative
  Derivative2 : Derivative
  Divide2 : Product  Inputs=*/
  Divide3 : Product  Inputs=*/
  Product{4..6,17..30} (17 alike) : Product
  Sqrt : Sqrt  SaturateOnIntegerOverflow=on
  Sqrt2 : Sqrt  SaturateOnIntegerOverflow=on
  Subsystem : Subsystem  Commented=on
  Sum1 : Sum  Inputs=+-|
  Sum10 : Sum  Inputs=|+-
  Sum{9,11..12,14} (4 alike) : Sum  Inputs=+|+
  Sum13 : Sum  Inputs=+|-
  Sum2 : Sum  Inputs=+++
  Sum7 : Sum  Inputs=+-|
  Switch{,1..3} (4 alike) : Switch  Criteria=u2 > Threshold
  lower_Vt1 : InportShadow  Port=2
  alpha_dot : Outport  Unit=rad/s
  beta_dot : Outport  Port=2
  wires:
  "u, v, w"/1 -> Demux/1
  Demux/1 -> Derivative/1, [u]  "u"
  Demux/2 -> Derivative1/1, [v]  "v"
  Demux/3 -> Derivative2/1, [w]  "w"
  [u] -> Product4/1, Product4/2
  [w] -> Product6/2, Product6/1
  [v] -> Product5/1, Product5/2
  Product4/1 -> Sum2/1
  Product6/1 -> Sum2/3
  Product5/1 -> Sum2/2
  Sum2/1 -> Sqrt/1
  Sqrt/1 -> [Vt]  "Vt"
  Derivative2/1 -> [w_dot]  "w_dot"
  Derivative/1 -> [u_dot]  "u_dot"
  Derivative1/1 -> [v_dot]  "v_dot"
  Sum7/1 -> Switch1/2
  [Vt] -> Sum7/1
  lower_Vt/1 -> Sum7/2
  [w_dot] -> Product17/1
  [u] -> Product17/2, Product26/2, Product26/1
  [w] -> Product27/1, Product27/2, Product18/1
  [u_dot] -> Product18/2
  Product26/1 -> Sum9/1
  Product27/1 -> Sum9/2
  Product17/1 -> Sum10/1
  Product18/1 -> Sum10/2
  Sum10/1 -> Divide2/1
  [u] -> Product28/1, Product28/2
  [w] -> Product29/2, Product29/1
  Product28/1 -> Sum11/1
  Product29/1 -> Sum11/2
  Sum11/1 -> Product30/2
  [v_dot] -> Product30/1
  [u_dot] -> Product19/2
  [w] -> Product20/1
  Product19/1 -> Sum12/1
  Product20/1 -> Sum12/2
  Sum12/1 -> Product21/1
  [u] -> Product19/1
  [w_dot] -> Product20/2
  [v] -> Product21/2
  Product30/1 -> Sum13/1
  Product21/1 -> Sum13/2
  Sum13/1 -> Divide3/1
  Product22/1 -> Sum14/1
  Product23/1 -> Sum14/2
  [u] -> Product22/2, Product22/1
  [w] -> Product23/2, Product23/1
  [Vt] -> Product25/1, Product25/2
  Product25/1 -> Product24/1
  Sum14/1 -> Sqrt2/1
  Sqrt2/1 -> Product24/2
  Switch/1 -> Divide2/2
  Sum9/1 -> Switch/2, Switch/1
  Constant2/1 -> Switch/3
  Switch2/1 -> Divide3/2
  Product24/1 -> Switch2/2, Switch2/1
  Constant3/1 -> Switch2/3
  Switch3/1 -> beta_dot/1
  Divide2/1 -> Switch1/1
  Switch1/1 -> alpha_dot/1
  Constant/1 -> Switch1/3
  Sum1/1 -> Switch3/2
  Constant1/1 -> Switch3/3
  Divide3/1 -> Switch3/1
  [Vt] -> Sum1/1
  lower_Vt1/1 -> Sum1/2

== system mainV03_52/Pilot Commands/Signal Builder ==
  Demux : Demux  Tag=STV Demux  Outputs=10
  FromWs : FromWorkspace  Tag=STV FromWs  VariableName=tuvar  SampleTime=0
      SigBuilderData=|
      | common.afterFinalStr = 'Extrapolate'
      | common.sampleTime = 0
      | dataSet.timeRange = [0 500]
      | dataSet.name = 'Group 1'
      | sbobj.Groups.Name = 'Group 1'
      | sbobj.Groups.Signals(1).Name = 'Roll'
      | sbobj.Groups.Signals(1).XData = [0 500]
      | sbobj.Groups.Signals(1).YData = [0 0]
      | sbobj.Groups.Signals(2).Name = 'Pitch'
      | sbobj.Groups.Signals(2).XData = [0 500]
      | sbobj.Groups.Signals(2).YData = [0 0]
      | sbobj.Groups.Signals(3).Name = 'Yaw'
      | sbobj.Groups.Signals(3).XData = [0 500]
      | sbobj.Groups.Signals(3).YData = [0 0]
      | sbobj.Groups.Signals(4).Name = 'Altitude'
      | sbobj.Groups.Signals(4).XData = [0 500]
      | sbobj.Groups.Signals(4).YData = [0 0]
      | sbobj.Groups.Signals(5).Name = 'Throttle1'
      | sbobj.Groups.Signals(5).XData = [0 500]
      | sbobj.Groups.Signals(5).YData = [0 0]
      | sbobj.Groups.Signals(6).Name = 'Throttle2'
      | sbobj.Groups.Signals(6).XData = [0 500]
      | sbobj.Groups.Signals(6).YData = [0 0]
      | sbobj.Groups.Signals(7).Name = 'Throttle3'
      | sbobj.Groups.Signals(7).XData = [0 500]
      | sbobj.Groups.Signals(7).YData = [0 0]
      | sbobj.Groups.Signals(8).Name = 'Throttle4'
      | sbobj.Groups.Signals(8).XData = [0 500]
      | sbobj.Groups.Signals(8).YData = [0 0]
      | sbobj.Groups.Signals(9).Name = 'Throttle5'
      | sbobj.Groups.Signals(9).XData = [0 500]
      | sbobj.Groups.Signals(9).YData = [0 0]
      | sbobj.Groups.Signals(10).Name = 'flightCondition'
      | sbobj.Groups.Signals(10).XData = [0 15 15 20 20 30 30 35 35 45 45 50 50 500]
      | sbobj.Groups.Signals(10).YData = [0 0 1 1 0 0 2.2 2.2 0 0 3 3 0 0]
      | sbobj.Groups.TimeRange = [0 500]
  Roll : Outport  Tag=STV Outport
  Pitch : Outport  Tag=STV Outport  Port=2
  Yaw : Outport  Tag=STV Outport  Port=3
  Altitude : Outport  Tag=STV Outport  Port=4
  Throttle1 : Outport  Tag=STV Outport  Port=5
  Throttle2 : Outport  Tag=STV Outport  Port=6
  Throttle3 : Outport  Tag=STV Outport  Port=7
  Throttle4 : Outport  Tag=STV Outport  Port=8
  Throttle5 : Outport  Tag=STV Outport  Port=9
  flightCondition : Outport  Tag=STV Outport  Port=10
  wires:
  FromWs/1 -> Demux/1
  Demux/1 -> Roll/1
  Demux/2 -> Pitch/1
  Demux/3 -> Yaw/1
  Demux/4 -> Altitude/1
  Demux/5 -> Throttle1/1
  Demux/6 -> Throttle2/1
  Demux/7 -> Throttle3/1
  Demux/8 -> Throttle4/1
  Demux/9 -> Throttle5/1
  Demux/10 -> flightCondition/1

== system mainV03_52/Sensors/Feedthrough Sensors ==
  States : Inport  OutDataTypeStr=Bus: plantDataBus
  Environment : Inport  Port=2  OutDataTypeStr=Bus: envDataBus
  Bus Creator2 : BusCreator  Inputs='LLAMeas','X_nedMeas','VearthMeas','AccelMeas_body','OmegaMeas_body','DCMMeas_body_earth','EulerMeas','VaeroMeas_body','alphaMeas','betaMeas','CGMeas','remainingCapacityMeas'  OutDataTypeStr=Bus: SensorsBus  NonVirtualBus=on
  CPU : Subsystem
  Environment_1 : InportShadow  Port=2  OutDataTypeStr=Bus: envDataBus
  GPS : Subsystem
  IMU : Subsystem
  Pitot : Subsystem
  Veleta : Subsystem
  Sensors : Outport  OutDataTypeStr=Bus: SensorsBus
  wires:
  Environment/1 -> IMU/2(Environment)
  IMU/4(EulerMeas) -> Bus Creator2/7  "EulerMeas"
  Bus Creator2/1 -> Sensors/1  "Sensors"
  CPU/1(CGMeas) -> Bus Creator2/11  "CGMeas"
  GPS/2(X_nedMeas) -> Bus Creator2/2  "X_nedMeas"
  States/1 -> IMU/1(States), GPS/1(States), Pitot/1(States), CPU/1(States), Veleta/1(States)
  IMU/2(OmegaMeas_body) -> Bus Creator2/5  "OmegaMeas_body"
  IMU/1(AccelMeas_body) -> Bus Creator2/4  "AccelMeas_body"
  GPS/1(LLAMeas) -> Bus Creator2/1  "LLAMeas"
  Veleta/1(alphaMeas) -> Bus Creator2/9  "alphaMeas"
  Environment_1/1 -> Pitot/2(Environment)
  Veleta/2(betaMeas) -> Bus Creator2/10  "betaMeas"
  Pitot/1(VaeroMeas_body) -> Bus Creator2/8  "VaeroMeas_body"
  CPU/2(remainingCapacityMeas) -> Bus Creator2/12  "remainingCapacityMeas"
  GPS/3(VearthMeas) -> Bus Creator2/3  "VearthMeas"
  IMU/3(DCMMeas_body_earth) -> Bus Creator2/6  "DCMMeas_body_earth"

== system mainV03_52/Sensors/Noisy Sensors ==
  States : Inport  OutDataTypeStr=Bus: plantDataBus
  Environment : Inport  Port=2  OutDataTypeStr=Bus: envDataBus
  Bus Creator2 : BusCreator  Inputs='LLAMeas','X_nedMeas','VearthMeas','AccelMeas_body','OmegaMeas_body','DCMMeas_body_earth','EulerMeas','VaeroMeas_body','alphaMeas','betaMeas','CGMeas','remainingCapacityMeas'  OutDataTypeStr=Bus: SensorsBus  NonVirtualBus=on
  CPU (Feedthough) : Subsystem
  Environment_1 : InportShadow  Port=2  OutDataTypeStr=Bus: envDataBus
  GPS (Feedthough) : Subsystem
  IMU : Subsystem
  Pitot (Feedthough) : Subsystem
  Veleta (Feedthough) : Subsystem
  Sensors : Outport  OutDataTypeStr=Bus: SensorsBus
  wires:
  Environment/1 -> IMU/2(Environment)
  IMU/4(EulerMeas) -> Bus Creator2/7  "EulerMeas"
  Bus Creator2/1 -> Sensors/1  "Sensors"
  CPU (Feedthough)/1(CGMeas) -> Bus Creator2/11  "CGMeas"
  GPS (Feedthough)/2(X_nedMeas) -> Bus Creator2/2  "X_nedMeas"
  States/1 -> GPS (Feedthough)/1(States), IMU/1(States), Pitot (Feedthough)/1(States), CPU (Feedthough)/1(States), Veleta (Feedthough)/1(States)
  IMU/2(OmegaMeas_body) -> Bus Creator2/5  "OmegaMeas_body"
  IMU/1(AccelMeas_body) -> Bus Creator2/4  "AccelMeas_body"
  GPS (Feedthough)/1(LLAMeas) -> Bus Creator2/1  "LLAMeas"
  Veleta (Feedthough)/1(alphaMeas) -> Bus Creator2/9  "alphaMeas"
  Environment_1/1 -> Pitot (Feedthough)/2(Environment)
  Veleta (Feedthough)/2(betaMeas) -> Bus Creator2/10  "betaMeas"
  Pitot (Feedthough)/1(VaeroMeas_body) -> Bus Creator2/8  "VaeroMeas_body"
  CPU (Feedthough)/2(remainingCapacityMeas) -> Bus Creator2/12  "remainingCapacityMeas"
  GPS (Feedthough)/3(VearthMeas) -> Bus Creator2/3  "VearthMeas"
  IMU/3(DCMMeas_body_earth) -> Bus Creator2/6  "DCMMeas_body_earth"

== system mainV03_52/Visualization/Airspeed Indicator ==

== system mainV03_52/Visualization/Altimeter ==

== system mainV03_52/Visualization/Artificial Horizon ==

== system mainV03_52/Visualization/Axes to VR Axes ==
  Xe : Inport
  Concatenate : Concatenate  NumInputs=3
  Constant : Constant  Value=1.01
  Demux : Demux  Outputs=3
  Sum : Sum  Inputs=|++
  rad-->deg : Gain  Gain=-1  SaturateOnIntegerOverflow=on  OutDataTypeStr=Inherit: Same as input  ParamDataTypeStr=Inherit: Same as input
  rad-->deg1 : Gain  Gain=-1  SaturateOnIntegerOverflow=on  OutDataTypeStr=Inherit: Same as input  ParamDataTypeStr=Inherit: Same as input
  Xe VR : Outport
  wires:
  Xe/1 -> Demux/1
  Concatenate/1 -> Xe VR/1
  rad-->deg1/1 -> Concatenate/2
  rad-->deg/1 -> Concatenate/1
  Demux/1 -> Concatenate/3
  Demux/2 -> rad-->deg/1
  Constant/1 -> Sum/2
  Demux/3 -> Sum/1
  Sum/1 -> rad-->deg1/1

== system mainV03_52/Visualization/Climb Rate Indicator ==

== system mainV03_52/Visualization/Half Gauge ==

== system mainV03_52/Visualization/Heading Indicator ==
